simulink model "OneSmartTankMod"  (R2020a)
settings: Solver=VariableStepAuto  StartTime=0.0  StopTime=100  RelTol=1e-3
libraries: mpclib x1, simulink x1
settings Model: Creator=lydialagorga  LastModifiedBy=lydialagorga

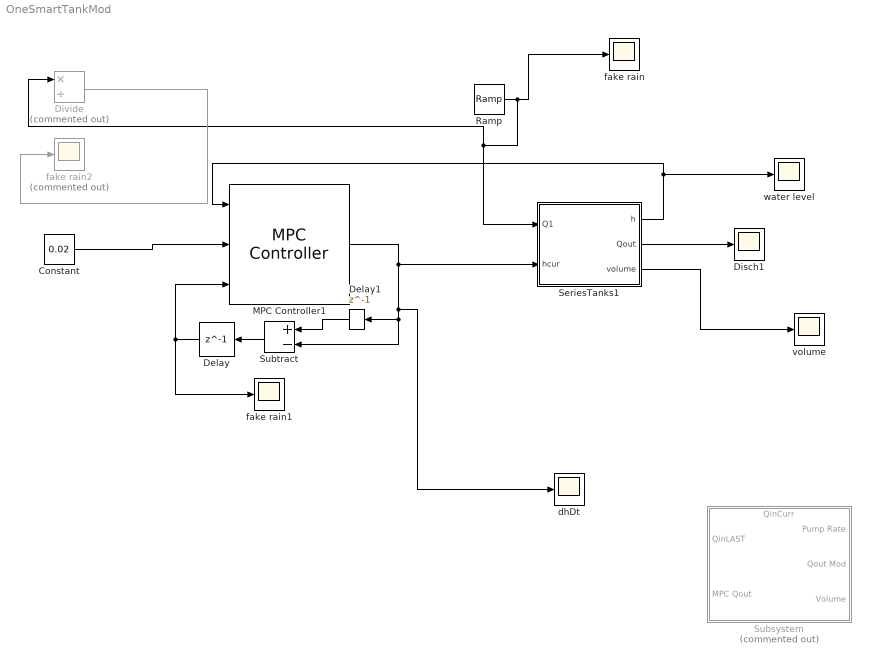
== system OneSmartTankMod ==
  Constant : Constant  Value=0.02
  Delay : Delay  DelayLength=1  InitialCondition=0
  Delay1 : Delay  DelayLength=1  InitialCondition=0
  Disch1 : Scope
  Divide : Product  Commented=on  Inputs=*/
  MPC Controller1 : mpclib/MPC Controller  SCDEnableBlockLinearizationSpecification=on  mpcobj=tankMPCobj  is_multiple=0  enable_value=0  return_u0=off  updateMPCinCallerWorkspace=on  md_inport=on  mv_inport=off  uref_inport=off  return_cost=off  return_mvseq=off  return_qpstatus=off  return_xseq=off  return_state=off  return_ovseq=off  state_inport=off  umin_inport=off  umax_inport=off  ymin_inport=off  ymax_inport=off  cc_inport=off  ywt_inport=off  uwt_inport=off  duwt_inport=off  rhoeps_inport=off  pm_inport=off  MaximumP=10  HorizonChoice=FixedHorizon  n_ts=1  n_p=10  n_mv=1  n_md=1  n_ud=0  n_mo=1  n_uo=0  BlockDataType=double  SampleTimeInherited=off  switch_inport=off
  Ramp : simulink/Sources/Ramp  slope=.2  start=5  InitialOutput=0
  SeriesTanks1 : Subsystem
  Subsystem : Subsystem  Commented=on
      settings: PortSchema="{\"entries\":[{\"content\":{\"sides\":[{\"content\":{\"connectorIds\":[\"In1\",\"In2\"]},\"type\":\"ConnectorPlacement.EquallySpacedRectSide\",\"uuid\":\"2e541fee-425f-42c5-8525-f22b933c6585\"},{\"content\":{\"connectorIds\":[\"Out1\",\"Out2\",\"Out3\"],\"side\":\"RIGHT\"},\"type\":\"ConnectorPlacement.EquallySpacedRectSide\",\"uuid\":\"dcba341a-88c3-4351-8c35-125a68807492\"},{\"content\":{\"connectorIds\":[\"In3\"],\"side\":\"TOP\"},\"type\":\"ConnectorPlacement.EquallySpacedRectSide\",\"uuid\":\"570c780b-565a-4e39-bb60-7f4dee45265d\"}]},\"type\":\"ConnectorPlacement.EquallySpacedConnector\",\"uuid\":\"11f8bf81-3cd8-4732-ae0c-3bac6e33cf31\"}],\"packageUris\":[\"http://schema.mathworks.com/mf0/Connector/19700101\"],\"version\":\"1.0\"}"
  Subtract : Sum  Inputs=+-
  dhDt : Scope
  fake rain : Scope
  fake rain1 : Scope
  fake rain2 : Scope  Commented=on
  volume : Scope
  water level : Scope
  wires:
  Ramp/1 -> SeriesTanks1/1(Q1), Divide/1, fake rain/1
  MPC Controller1/1 -> SeriesTanks1/2(hcur), Delay1/1, Subtract/2, dhDt/1
  SeriesTanks1/1(h) -> water level/1, MPC Controller1/1
  SeriesTanks1/2(Qout) -> Disch1/1
  Divide/1 -> fake rain2/1
  Subtract/1 -> Delay/1
  Delay/1 -> MPC Controller1/3, fake rain1/1
  SeriesTanks1/3(volume) -> volume/1
  Delay1/1 -> Subtract/1
  Constant/1 -> MPC Controller1/2

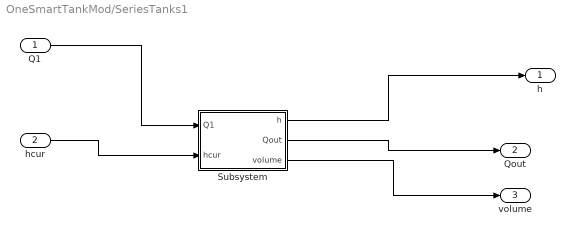
== system OneSmartTankMod/SeriesTanks1 ==
  Q1 : Inport
  hcur : Inport  Port=2
  Subsystem : Subsystem
      settings: PermitHierarchicalResolution=None
  h : Outport
  Qout : Outport  Port=2
  volume : Outport  Port=3
  wires:
  Q1/1 -> Subsystem/1(Q1)
  Subsystem/1(h) -> h/1
  Subsystem/2(Qout) -> Qout/1
  hcur/1 -> Subsystem/2(hcur)
  Subsystem/3(volume) -> volume/1

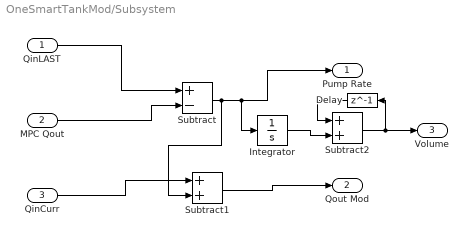
== system OneSmartTankMod/Subsystem ==
  QinLAST : Inport
  MPC Qout : Inport  Port=2
  QinCurr : Inport  Port=3
  Delay : Delay  DelayLength=1  InitialCondition=0
  Integrator : Integrator
  Subtract : Sum  Inputs=+-
  Subtract1 : Sum
  Subtract2 : Sum
  Pump Rate : Outport  OutMin=0
  Qout Mod : Outport  Port=2  OutMin=0
  Volume : Outport  Port=3  OutMin=0
  wires:
  MPC Qout/1 -> Subtract/2
  QinLAST/1 -> Subtract/1
  QinCurr/1 -> Subtract1/1
  Subtract1/1 -> Qout Mod/1
  Subtract/1 -> Integrator/1, Pump Rate/1, Subtract1/2
  Subtract2/1 -> Delay/1, Volume/1
  Delay/1 -> Subtract2/1
  Integrator/1 -> Subtract2/2

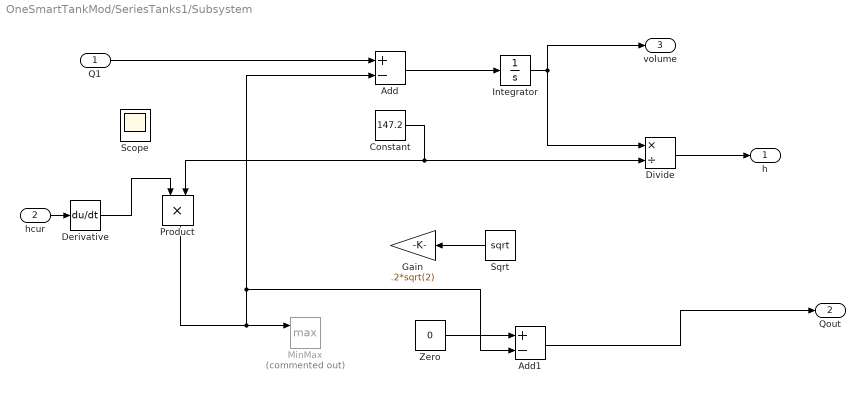
== system OneSmartTankMod/SeriesTanks1/Subsystem ==
  Q1 : Inport
  hcur : Inport  Port=2
  Add : Sum  Inputs=+-
  Add1 : Sum  Inputs=+-
  Constant : Constant  Value=147.2
  Derivative : Derivative
  Divide : Product  Inputs=*/
  Gain : Gain  Gain=.2*sqrt(2)
  Integrator : Integrator  LimitOutput=on  UpperSaturationLimit=100  LowerSaturationLimit=0
  MinMax : MinMax  Commented=on  Function=max  Inputs=2
  Product : Product
  Scope : Scope
  Sqrt : Sqrt  SaturateOnIntegerOverflow=on
  Zero : Constant  Value=0  OutDataTypeStr=Inherit: Inherit via back propagation
  h : Outport  OutMin=0
  Qout : Outport  Port=2  OutMin=0  OutMax=100
  volume : Outport  Port=3  OutMin=0
  wires:
  Sqrt/1 -> Gain/1
  Add/1 -> Integrator/1
  Q1/1 -> Add/1
  Integrator/1 -> Divide/1, volume/1
  Constant/1 -> Divide/2, Product/2
  Divide/1 -> h/1
  Product/1 -> Add/2, Add1/2, MinMax/1
  hcur/1 -> Derivative/1
  Derivative/1 -> Product/1
  Zero/1 -> Add1/1
  Add1/1 -> Qout/1
